simulink model "siWDqudong_FAN_MPC"  (R2024b)
settings: Solver=ode4  StartTime=0.0  StopTime=30  FixedStep=0.0005  RelTol=1e-3
undefined symbols (not defined in the file): MotorData, Q_beta_tune, Q_yaw_tune, R_alloc_tune, R_rate_tune, Road_Curvature_Map, Road_Mu_Map, Sim_Mu_Set, Sim_Vx_Set, Target_Speed_Map, W_util_tune
libraries: Solver_SF x1
(part 2 of 3)

== matlab function siWDqudong_FAN_MPC/Subsystem1/MATLAB Function2 ==
  settings: updateMethod=DISCRETE
  data: T_fl input; P_total_kW output; T_fr input; T_rl input; T_rr input; w_fl input; w_fr input; w_rl input; w_rr input; Map_Spd input; Map_Trq input; Map_Eff input; dt input; is_reset input; E_total_kWh output; P_avg_kW output
function [P_total_kW, E_total_kWh, P_avg_kW] = Calc_Energy_Internal_Map(...
    T_fl, T_fr, T_rl, T_rr, ...       
    w_fl, w_fr, w_rl, w_rr, ...       
    Map_Spd, Map_Trq, Map_Eff, ...    
    dt, is_reset)                     
%#codegen
% =========================================================================
% 全工况能耗计算器 v11.1 (最终版)
% [核心特性]
% 1. 完整覆盖驱动与制动回收双象限查表 (原样保留负转矩传入查表)。
% 2. 包含 35% 低扭效率兜底机制，避免除零或无穷大功率奇点，更贴合实际物理下限。
% 3. 包含车规级制动回收保护：低速 (<5 rad/s) 与低效 (<20%) 区间强制切断。
% =========================================================================
    persistent E_accumulated_J Total_Time_s
    if isempty(E_accumulated_J) || is_reset
        E_accumulated_J = 0;
        Total_Time_s = 0;
    end
    
    T_vec = [double(T_fl), double(T_fr), double(T_rl), double(T_rr)];
    w_vec = [double(w_fl), double(w_fr), double(w_rl), double(w_rr)];
    
    % --- ★ 轮毂电机物理与工程参数 ★ ---
    i_gear = 1.0; % 直驱轮毂电机减速比
    P_base_loss_W = 150.0; % 逆变器与控制器的基础待机损耗 (W)
    
    vec_x_rad = double(Map_Spd); 
    vec_y_nm  = double(Map_Trq); 
    mat_eff   = double(Map_Eff)';
    
    P_elec_W_vec = zeros(1, 4);
    
    for i = 1:4
        T_wheel = T_vec(i);     
        w_wheel_rads = w_vec(i);     
        
        % 1. 计算电机端工况
        % ★ 核心：速度取绝对值，扭矩保留正负号，以精确匹配四象限 Map 表！
        T_motor = T_wheel / i_gear; 
        w_motor_rads = abs(w_wheel_rads) * i_gear; 
        
        % 计算轮端机械功率 (驱动时为正，制动反拖时为负)
        P_mech_wheel = T_wheel * w_wheel_rads; 
        
        % 2. 极端静止/空转工况拦截
        if abs(w_wheel_rads) < 1.0
            % 车辆基本停稳，电机停止输出，彻底切断电能消耗
            P_elec = 0; 
        elseif abs(T_wheel) < 3.0 
            % 车辆滑行或该轮被上层分配 0 扭矩，仅消耗基础待机电量
            P_elec = P_base_loss_W; 
        else
            % 3. 正常工况：查表获取当前效率
            eff_raw = manual_interp2(vec_x_rad, vec_y_nm, mat_eff, w_motor_rads, T_motor);
            
            % 4. 驱动与制动能量流向计算
            if P_mech_wheel > 0
                % =========================================================
                % 【驱动耗电模式】
                % 引入 35% 的工程效率兜底，防止极低扭矩时的能耗被数学奇点无限放大
                % 消耗电功率 = (机械功率 / 效率) + 基础待机功耗
                % =========================================================
                eff_final = max(eff_raw, 0.35); 
                P_elec = (P_mech_wheel / eff_final) + P_base_loss_W;
                
            else
                % =========================================================
                % 【制动回收模式 (Regenerative Braking)】
                % P_mech_wheel 为负值
                % =========================================================
                if eff_raw < 0.20 || w_motor_rads < 5.0 
                    % 工程保护机制：低速域或极低效率域，强行切断激磁回收
                    % 避免开关损耗大于回收收益的现象
                    P_elec = P_base_loss_W; 
                else
                    % 物理能量守恒：
                    % 负的机械功率 * 效率 = 缩水的负电功率 (代表实际回充至母线的电量)
                    % 加上正的待机功耗，进一步减少了最终充入电池的能量
                    P_elec = (P_mech_wheel * eff_raw) + P_base_loss_W; 
                end
            end
        end
        % 记录单个车轮的总电功率
        P_elec_W_vec(i) = P_elec;
    end
    
    % --- 5. 整车能耗累加与统计 ---
    P_total_W = sum(P_elec_W_vec);       % 整车瞬时总功率 (W)
    P_total_kW = P_total_W / 1000;       % 整车瞬时总功率 (kW)
    
    % 焦耳积分 (J = W * s)
    E_accumulated_J = E_accumulated_J + P_total_W * double(dt);
    Total_Time_s = Total_Time_s + double(dt);
    
    % 转换为 kWh (1 kWh = 3.6e6 J)
    E_total_kWh = E_accumulated_J / 3.6e6;
    
    % 计算全历程平均功率
    if Total_Time_s > 1e-3
        P_avg_kW = (E_accumulated_J / Total_Time_s) / 1000;
    else
        P_avg_kW = 0;
    end
end

% ==== 手写双线性插值函数 (Bilinear Interpolation) ====
function val = manual_interp2(X, Y, Z, xq, yq)
    % 边界钳位保护
    xq_c = max(min(xq, X(end)), X(1));
    yq_c = max(min(yq, Y(end)), Y(1));
    
    % 寻找 X 轴索引
    idx_x = 1;
    for k = 1:length(X)-1
        if xq_c >= X(k) && xq_c <= X(k+1), idx_x = k; break; end
    end
    
    % 寻找 Y 轴索引
    idx_y = 1;
    for k = 1:length(Y)-1
        if yq_c >= Y(k) && yq_c <= Y(k+1), idx_y = k; break; end
    end
    
    x1 = X(idx_x); x2 = X(idx_x+1);
    y1 = Y(idx_y); y2 = Y(idx_y+1);
    
    % 归一化局部坐标
    if abs(x2-x1)<1e-9, u=0; else, u=(xq_c-x1)/(x2-x1); end
    if abs(y2-y1)<1e-9, v=0; else, v=(yq_c-y1)/(y2-y1); end
    
    % 四点提取
    f11 = Z(idx_y,   idx_x);
    f21 = Z(idx_y,   idx_x+1);
    f12 = Z(idx_y+1, idx_x);
    f22 = Z(idx_y+1, idx_x+1);
    
    % 双线性加权
    val = (1-v)*((1-u)*f11 + u*f21) + v*((1-u)*f12 + u*f22);
    
    if isnan(val), val = 0.01; end
end

== matlab function siWDqudong_FAN_MPC/Subsystem1/MATLAB Function17 ==
  data: Vx input; r_d output; delta_f input; mu input; m input; lf input; lr input; K_s output; r_ideal output; Kf0 input; Kr0 input; g input; r_limit output
function [r_d, K_s, r_ideal, r_limit] = ReferenceYawRate(Vx, delta_f, mu, m, lf, lr, Kf0, Kr0, g)
% =========================================================================
% 参考横摆角速度生成 (鲁棒增强版)
% 修复内容：低速奇点保护、物理极限柔性化、输出平滑
% =========================================================================

    % 1. 参数默认值与保护
    if nargin < 9, g = 9.81; end
    
    % 输入数据维度清洗 (强制转为标量 double)
    Vx_in = double(Vx(1));
    delta_in = double(delta_f(1));
    mu_in = double(mu(1));

    % 速度方向与绝对值处理
    Vx_sign = sign(Vx_in);
    if Vx_sign == 0, Vx_sign = 1; end
    Vx_abs = abs(Vx_in);
    
    % 基础防除零保护 (计算模型用)
    Vx_safe = max(Vx_abs, 0.5); 

    % =====================================================================
    % 2. 计算稳态增益 (Steady State Gain)
    % =====================================================================
    K_s = m / (2 * (lf + lr)^2) * (lr/Kf0 - lf/Kr0);

    % =====================================================================
    % 3. 计算理想横摆角速度 (Linear 2DOF Model)
    % =====================================================================
    % 分母：1 + K * V^2
    denom = (lf + lr) * (1 + K_s * Vx_safe^2);
    
    if abs(denom) < 0.1
        r_ideal = 0;
    else
        % r_ideal = (Vx / L(1+KV^2)) * delta
        r_ideal = (Vx_safe / denom) * delta_in * Vx_sign; 
    end

    % =====================================================================
    % 4. 计算物理极限 (【关键修复点】)
    % =====================================================================
    % 原公式：Limit = 0.85 * mu * g / Vx
    % 问题：当车辆甩尾速度掉到 1m/s 时，Limit 会变成 0.85*0.8*9.8/1 = 6.6 rad/s (380度/秒)
    % 修复：计算极限时，假设速度至少为 5m/s (虚拟速度钳位)
    % 逻辑：低速时侧向加速度其实达不到 mu*g，因为离心力不够，所以这样限制更符合物理
    
    Vx_for_limit = max(Vx_abs, 5.0); 
    
    % 计算理论上限
    r_limit_val = 0.85 * mu_in * g / Vx_for_limit;
    
    % 【双重保险】增加一个绝对硬限幅 (例如 1.5 rad/s ≈ 85 deg/s)
    % 防止任何情况下的数值爆炸
    r_limit_val = min(r_limit_val, 1.5);

    % =====================================================================
    % 5. 柔性限幅 (Saturation)
    % =====================================================================
    if r_ideal > r_limit_val
        r_d_raw = r_limit_val;
    elseif r_ideal < -r_limit_val
        r_d_raw = -r_limit_val;
    else
        r_d_raw = r_ideal;
    end

    % =====================================================================
    % 6. 强力滤波 (平滑输出)
    % =====================================================================
    persistent rd_prev
    if isempty(rd_prev), rd_prev = 0; end
    
    % 滤波系数：0.05 代表非常强的滤波 (响应慢，但稳)，如果觉得滞后太大可改为 0.1
    alpha_filter = 0.05; 
    
    r_d_smooth = (1 - alpha_filter) * rd_prev + alpha_filter * r_d_raw;
    
    % 更新记忆
    rd_prev = r_d_smooth;

    % =====================================================================
    % 7. 输出类型转换
    % =====================================================================
    r_d = double(r_d_smooth);
    r_ideal = double(r_ideal);
    r_limit = double(r_limit_val);
    
end

== matlab function siWDqudong_FAN_MPC/Subsystem1/MATLAB Function15 ==
  data: Vx_cmd input; Vx_act_raw input; T_total output; Ax_cmd input; m input; g input; r_e input; Kp input; Ki input; dt input; is_reset input; T_ff output; T_fb output; delta_steering input; Mu_in input; Curv_in input; Beta_in input; SI_in input
function [T_total, T_ff, T_fb] = Calc_Total_Demand_Torque( ...
    Vx_cmd, Vx_act_raw, Ax_cmd, ...
    m, g, r_e, ...
    Kp, Ki, dt, is_reset, delta_steering, Mu_in, ...
    Curv_in, Beta_in, SI_in)
%#codegen
% Fixed-speed longitudinal torque demand for closed-loop BO.
% Safety remains enforced by physical torque limits and downstream
% stability constraints; the controller does not silently lower Vx_cmd.

    persistent Vx_act_f Mu_f steer_f T_prev T_int Risk_f initialized

    if isempty(Vx_act_f) || is_reset
        Vx_act_f = double(Vx_act_raw);
        Mu_f = max(0.15,double(Mu_in(1)));
        steer_f = abs(double(delta_steering));
        T_prev = 0.0;
        T_int = 0.0;
        Risk_f = 0.0;
        initialized = false;
    end

    if dt <= 1e-5
        dt = 0.01;
    end

    Vx_cmd_use = max(0.0,double(Vx_cmd));
    Vx_act_raw_use = max(0.0,double(Vx_act_raw));
    Ax_cmd_use = double(Ax_cmd);

    alpha_v = 0.08;
    alpha_mu = 0.03;
    alpha_st = 0.10;
    Vx_act_f = (1.0-alpha_v)*Vx_act_f + alpha_v*Vx_act_raw_use;
    Mu_raw = max(0.15,double(Mu_in(1)));
    Mu_f = (1.0-alpha_mu)*Mu_f + alpha_mu*Mu_raw;
    steer_f = (1.0-alpha_st)*steer_f + alpha_st*abs(double(delta_steering));

    Vx_act = Vx_act_f;
    Mu_est = Mu_f;

    kappa_abs = abs(double(Curv_in(1)));
    beta_abs = abs(double(Beta_in(1)));
    SI_val = double(SI_in(1));
    ay_req = Vx_act*Vx_act*kappa_abs;
    ay_lim = max(Mu_est*g,0.10);
    ay_ratio = ay_req/ay_lim;

    R_ay = clamp((ay_ratio-0.78)/0.15,0.0,1.0);
    R_beta = clamp((beta_abs-0.045)/0.035,0.0,1.0);
    R_SI = clamp((SI_val-0.65)/0.35,0.0,1.0);
    R_st = clamp((steer_f-0.030)/0.040,0.0,1.0);
    Raw_Risk = max([R_ay,0.8*R_beta,0.6*R_SI,0.4*R_st]);

    if Raw_Risk >= Risk_f
        alpha_risk = 0.18;
    else
        alpha_risk = 0.06;
    end
    Risk_f = (1.0-alpha_risk)*Risk_f + alpha_risk*Raw_Risk;
    Risk_long = clamp(Risk_f,0.0,1.0);

    % Road-load feedforward is evaluated at the commanded speed.  Blending
    % it toward measured speed creates positive feedback for underspeed and
    % caused the old V5 controller to keep losing torque as Vx fell.
    Vx_ff = Vx_cmd_use;
    Cd = 0.30;
    Af = 2.8;
    rho = 1.206;
    f_roll = 0.015;
    if abs(Vx_ff) > 0.2
        sgn_v = sign(Vx_ff);
    else
        sgn_v = 0.0;
    end
    F_aero = 0.5*rho*Cd*Af*Vx_ff*Vx_ff*sgn_v;
    F_roll = m*g*f_roll*sgn_v;
    F_acc = m*Ax_cmd_use;
    T_ff = (F_aero+F_roll+F_acc)*r_e;

    % Symmetric PI speed hold.  Risk is not allowed to disable positive
    % feedback; an infeasible fixed-speed condition must fail explicitly.
    e = Vx_cmd_use-Vx_act;
    deadband = 0.02;
    if e > deadband
        e_ctrl = e-deadband;
    elseif e < -deadband
        e_ctrl = e+deadband;
    else
        e_ctrl = 0.0;
    end

    Kp_use = max(double(Kp),0.0);
    Ki_use = max(double(Ki),0.0);
    T_int_old = T_int;
    T_int = clamp(T_int+Ki_use*e_ctrl*dt,-80.0,160.0);
    T_fb = Kp_use*e_ctrl+T_int;

    T_max_limit = 1500.0*(Mu_est/0.85);
    T_min_limit = -800.0*(Mu_est/0.85);
    if Risk_long > 0.28
        T_max_limit = max(160.0,0.82*T_max_limit);
    end

    T_cmd = T_ff+T_fb;
    T_sat = clamp(T_cmd,T_min_limit,T_max_limit);

    % Conditional integration prevents windup at the physical limits.
    if (T_cmd > T_max_limit && e_ctrl > 0.0) || ...
       (T_cmd < T_min_limit && e_ctrl < 0.0)
        T_int = T_int_old;
        T_fb = Kp_use*e_ctrl+T_int;
        T_cmd = T_ff+T_fb;
        T_sat = clamp(T_cmd,T_min_limit,T_max_limit);
    end

    % Initialize at the physical feedforward demand instead of ramping from
    % zero torque while the vehicle already starts at the target speed.
    if ~initialized || is_reset
        T_prev = T_sat;
        initialized = true;
    end

    if Risk_long > 0.28
        dT_up_rate = 500.0;
        dT_dn_rate = 800.0;
    else
        dT_up_rate = 800.0;
        dT_dn_rate = 800.0;
    end
    dT_up = dT_up_rate*dt;
    dT_dn = dT_dn_rate*dt;
    dT = T_sat-T_prev;
    if dT > dT_up
        T_total = T_prev+dT_up;
    elseif dT < -dT_dn
        T_total = T_prev-dT_dn;
    else
        T_total = T_sat;
    end
    T_prev = T_total;
end

function y = clamp(x,lo,hi)
    y = max(min(x,hi),lo);
end

== matlab function siWDqudong_FAN_MPC/Subsystem1/MATLAB Function18 ==
  settings: updateMethod=DISCRETE  sampleTime=0.01
  data: Vx_target_input input; Vx_safe_cmd output; dt input; Ax_cmd_final output
function [Vx_safe_cmd, Ax_cmd_final] = Constant_Speed_Planner(Vx_target_input, dt)
    % Constant_Speed_Planner
    % 功能：生成恒定目标车速和加速度指令
    
    % ================= 1. 数据预处理 (维度安全锁) =================
    % 强制转换为 double
    temp_v = double(Vx_target_input);
    
    % 【关键修改】防止输入变成向量 [4x1]
    % 如果输入是向量，取第一个元素或取平均值，确保输出是标量 [1x1]
    if numel(temp_v) > 1
        target_v = mean(temp_v); % 或者 target_v = temp_v(1);
    else
        target_v = temp_v;
    end
    
    % 限幅保护
    if isnan(target_v)
        target_v = 0;
    end
    target_v = max(target_v, 0); 

    % ================= 2. 指令生成 =================
    Vx_safe_cmd = target_v;
    
    % 理论加速度设为0
    Ax_cmd_final = 0; 
    
    % (可选) 如果未来想用 dt 做平滑处理，可以在这里写逻辑
    % 目前 dt 虽然未被使用，但保留在输入端口没问题，不会报错
end

== matlab function siWDqudong_FAN_MPC/Subsystem1/MATLAB Function19 ==
  data: Beta input; Beta_dot input; Vx input; mu input; delta_f input; SI_Out output
function SI_Out = fcn_Calculate_SI(Beta, Beta_dot, Vx, mu, delta_f)
%#codegen
%
% ================================================================
% TVT Phase-Plane Stability Index
% 与原始 TVT_PhasePlane_Deliverable_2026-09-06 中
% TVT_StableBoundary.m 的联合拟合模型严格一致
%
% Inputs:
%   Beta      - 质心侧偏角 beta [rad]
%   Beta_dot  - 质心侧偏角速度 beta_dot [rad/s]
%   Vx        - 车辆纵向速度 [m/s]
%   mu        - 路面附着系数 [-]
%   delta_f   - 前轮转角 [rad]
%
% Output:
%   SI_Out    - 相平面稳定性指标
%
% 原始定义：
%
%   lower <= beta + A*beta_dot <= upper
%
%   center = k * delta_f
%   lower  = center - B
%   upper  = center + B
%
%   SI = abs(beta + A*beta_dot - center) / B
%
%   SI <= 1 : 位于拟合稳定区域内部
%   SI >  1 : 超出拟合稳定边界
%
% ================================================================


%% ================================================================
% 1. 原始联合拟合输入标准化参数
% ================================================================

MuCenter = 0.588775510204082;
MuScale  = 0.199025047136673;

VCenter  = 19.530612244898;
VScale   = 6.17488880067328;


%% ================================================================
% 2. 标准化输入
% ================================================================

mu_s = (mu - MuCenter) / MuScale;
v_s  = (Vx - VCenter) / VScale;


%% ================================================================
% 3. 原始联合拟合：A(V,mu)
%
% X6 =
% [1,
%  mu_s,
%  v_s,
%  mu_s^2,
%  mu_s*v_s,
%  v_s^2]
%
% 系数完全来自：
% phase_joint_fit_coefficients.csv
% ================================================================

a0 =  0.161558225154477;
a1 = -0.0467387963496101;
a2 =  0.0117445583275526;
a3 =  0.0102656813192654;
a4 =  0.000166133673754782;
a5 =  0.012427427190128;

A = ...
      a0 ...
    + a1 * mu_s ...
    + a2 * v_s ...
    + a3 * mu_s * mu_s ...
    + a4 * mu_s * v_s ...
    + a5 * v_s * v_s;


%% ================================================================
% 4. 原始联合拟合：半宽 B(V,mu)
%
% X9 =
% [1,
%  mu_s,
%  v_s,
%  mu_s^2,
%  mu_s*v_s,
%  v_s^2,
%  mu_s^2*v_s,
%  mu_s*v_s^2,
%  mu_s^2*v_s^2]
%
% 系数完全来自：
% phase_joint_fit_coefficients.csv
% ================================================================

b0 =  0.109427337783177;
b1 =  0.0142990282924419;
b2 = -0.0381098451846239;
b3 =  0.00694057641920019;
b4 = -0.00200034946269806;
b5 =  0.0266201953812123;
b6 =  0.0105740728277829;
b7 = -0.00475737528037003;
b8 = -0.00798511539344205;

mu_s2 = mu_s * mu_s;
v_s2  = v_s  * v_s;

B = ...
      b0 ...
    + b1 * mu_s ...
    + b2 * v_s ...
    + b3 * mu_s2 ...
    + b4 * mu_s * v_s ...
    + b5 * v_s2 ...
    + b6 * mu_s2 * v_s ...
    + b7 * mu_s * v_s2 ...
    + b8 * mu_s2 * v_s2;


%% ================================================================
% 5. 原始联合拟合：中心位置 C(delta_f)
%
% 原始模型：
% center = ShiftK * delta_rad
% ================================================================

ShiftK = 1.00429232124377;

center = ShiftK * delta_f;


%% ================================================================
% 6. 原始相平面稳定性指标
%
% 与 TVT_StableBoundary.m 完全相同：
%
% SI = abs(beta + A*beta_dot - center)/B
% ================================================================

SI_Out = abs(Beta + A * Beta_dot - center) / B;

end

== matlab function siWDqudong_FAN_MPC/Subsystem1/MATLAB Function23 ==
  data: Fy_fl input; Cf_eq output; Fy_fr input; Fy_rl input; Fy_rr input; Alpha_fl input; Alpha_fr input; Alpha_rl input; Alpha_rr input; Cf0 input; Cr0 input; Cr_eq output; Mu_Current input
function [Cf_eq, Cr_eq] = fcn_Calc_Equivalent_Stiffness_Filtered(...
    Fy_fl, Fy_fr, Fy_rl, Fy_rr, ...
    Alpha_fl, Alpha_fr, Alpha_rl, Alpha_rr, ...
    Cf0, Cr0, Mu_Current) % ★ 新增输入: 当前路面附着 Mu_Current
% =========================================================================
% 非线性侧偏刚度估算模块 (前馈预警 + 实时估算混合版)
% =========================================================================
    persistent Cf_prev Cr_prev
    if isempty(Cf_prev)
        Cf_prev = Cf0 * 2; 
        Cr_prev = Cr0 * 2;
    end
    
    % =====================================================================
    % ★ 核心新增：基于附着系数的前馈压制 (Feed-forward Penalty) ★
    % 当车进入冰雪路面时，不用等侧滑发生，直接从物理极限上压低标称刚度！
    % =====================================================================
    mu_nominal = 0.85;
    mu_real = max(min(double(Mu_Current(1)), 1.0), 0.1);
    % 计算附着衰减系数
    mu_ratio = mu_real / mu_nominal; 
    
    % 前馈修正后的基础刚度 (冰面上基础刚度会瞬间掉下来)
    Cf_base_dyn = (Cf0 * 2) * mu_ratio;
    Cr_base_dyn = (Cr0 * 2) * mu_ratio;

    Fy_front_sum = abs(Fy_fl + Fy_fr);
    Fy_rear_sum  = abs(Fy_rl + Fy_rr);
    Alpha_front_avg = abs(Alpha_fl + Alpha_fr) / 2.0;
    Alpha_rear_avg  = abs(Alpha_rl + Alpha_rr) / 2.0;
    
    alpha_deadzone = 0.0087; 
    
    if Alpha_front_avg > alpha_deadzone
        Cf_inst = Fy_front_sum / Alpha_front_avg;
    else
        Cf_inst = Cf_base_dyn; % 小角度时用前馈修正的刚度
    end
    
    if Alpha_rear_avg > alpha_deadzone
        Cr_inst = Fy_rear_sum / Alpha_rear_avg;
    else
        Cr_inst = Cr_base_dyn; % 小角度时用前馈修正的刚度
    end
    
    % ★ 限幅逻辑也要跟着附着系数前馈一起下降 ★
    Cf_min = Cf_base_dyn * 0.3;  Cf_max = Cf_base_dyn * 1.5;
    Cr_min = Cr_base_dyn * 0.3;  Cr_max = Cr_base_dyn * 1.5;
    
    Cf_target = max(min(Cf_inst, Cf_max), Cf_min);
    Cr_target = max(min(Cr_inst, Cr_max), Cr_min);
    
    % 为了应对附着突变，如果是从高附着到低附着（刚度需要暴降），加快滤波速度
    if Cf_target < Cf_prev
        lambda = 0.3; % 变滑了，降刚度要快！(0.05太慢了)
    else
        lambda = 0.05; % 恢复抓地力，慢慢升
    end
    
    Cf_filt = (1 - lambda) * Cf_prev + lambda * Cf_target;
    Cr_filt = (1 - lambda) * Cr_prev + lambda * Cr_target;
    
    Cf_prev = Cf_filt; Cr_prev = Cr_filt;
    Cf_eq = Cf_filt; Cr_eq = Cr_filt;
end

== matlab function siWDqudong_FAN_MPC/Subsystem1/MATLAB Function5 ==
  data: Vx input; Sx_fr output; Vy input; r input; omega_fr input; delta_f input; lf input; twf input; Re input; Sy_fr output; Vsx_fr output; Vsy_fr output
function [Sx_fr, Sy_fr, Vsx_fr, Vsy_fr] = Cal_UniTire_FullData_FR(Vx, Vy, r, omega_fr, delta_f, lf, twf, Re)
% Cal_UniTire_FullData_FR - 右前轮全参数计算

    % === 1. 运动学解算 ===
    % 右前轮：纵向 +lf, 横向 -twf/2 (右侧)
    % Vx修正: 右侧轮在左转(r>0)时线速度增加，所以是 + r*(twf/2)
    V_cx = Vx + r * (twf / 2);  
    V_cy = Vy + r * lf;         

    % === 2. 坐标旋转 (车轮坐标系) ===
    cos_d = cos(delta_f);
    sin_d = sin(delta_f);
    
    V_long = V_cx * cos_d + V_cy * sin_d;
    V_lat  = -V_cx * sin_d + V_cy * cos_d;

    % === 3. 计算滑移速度 (能耗用) ===
    V_wheel = omega_fr * Re;
    Vsx_fr = V_wheel - V_long; % 纵向滑移速度
    Vsy_fr = V_lat;            % 侧向滑移速度

    % === 4. 计算滑移率 (轮胎模型用) ===
    V_long_safe = max(abs(V_long), 1.0); 
    
    Sx_fr = Vsx_fr / V_long_safe;
    Sy_fr = -Vsy_fr / V_long_safe; % UniTire定义带负号

    % === 5. 限幅 ===
    Sx_fr = max(min(Sx_fr, 1.5), -1.5);
    Sy_fr = max(min(Sy_fr, 1.5), -1.5);
end

== matlab function siWDqudong_FAN_MPC/Subsystem1/MATLAB Function6 ==
  data: Vx input; Sx_rl output; Vy input; r input; omega_rl input; lr input; twr input; Re input; Sy_rl output; Vsx_rl output; Vsy_rl output
function [Sx_rl, Sy_rl, Vsx_rl, Vsy_rl] = Cal_UniTire_FullData_RL(Vx, Vy, r, omega_rl, lr, twr, Re)
% Cal_UniTire_FullData_RL - 左后轮全参数计算
% 注意：后轮默认无转向角 (delta = 0)

    % === 1. 运动学解算 ===
    % 左后轮：纵向 -lr, 横向 +twr/2 (左侧)
    % Vcx: 左侧减去横摆分量
    % Vcy: 后轴减去横摆分量 (Vy - r*lr)
    V_cx = Vx - r * (twr / 2);  
    V_cy = Vy - r * lr;         

    % === 2. 坐标旋转 (后轮 delta=0) ===
    % cos(0)=1, sin(0)=0，其实就是不用旋转
    V_long = V_cx;
    V_lat  = V_cy;

    % === 3. 计算滑移速度 (能耗用) ===
    V_wheel = omega_rl * Re;
    Vsx_rl = V_wheel - V_long; 
    Vsy_rl = V_lat;            

    % === 4. 计算滑移率 (轮胎模型用) ===
    V_long_safe = max(abs(V_long), 1.0); 
    
    Sx_rl = Vsx_rl / V_long_safe;
    Sy_rl = -Vsy_rl / V_long_safe;

    % === 5. 限幅 ===
    Sx_rl = max(min(Sx_rl, 1.5), -1.5);
    Sy_rl = max(min(Sy_rl, 1.5), -1.5);
end

== matlab function siWDqudong_FAN_MPC/Subsystem1/MATLAB Function7 ==
  data: Vx input; Sx_rr output; Vy input; r input; omega_rr input; lr input; twr input; Re input; Sy_rr output; Vsx_rr output; Vsy_rr output
function [Sx_rr, Sy_rr, Vsx_rr, Vsy_rr] = Cal_UniTire_FullData_RR(Vx, Vy, r, omega_rr, lr, twr, Re)
% Cal_UniTire_FullData_RR - 右后轮全参数计算
% 注意：后轮默认无转向角 (delta = 0)

    % === 1. 运动学解算 ===
    % 右后轮：纵向 -lr, 横向 -twr/2 (右侧)
    % Vcx: 右侧加上横摆分量
    % Vcy: 后轴减去横摆分量
    V_cx = Vx + r * (twr / 2);  
    V_cy = Vy - r * lr;         

    % === 2. 坐标旋转 (后轮 delta=0) ===
    V_long = V_cx;
    V_lat  = V_cy;

    % === 3. 计算滑移速度 (能耗用) ===
    V_wheel = omega_rr * Re;
    Vsx_rr = V_wheel - V_long; 
    Vsy_rr = V_lat;            

    % === 4. 计算滑移率 (轮胎模型用) ===
    V_long_safe = max(abs(V_long), 1.0); 
    
    Sx_rr = Vsx_rr / V_long_safe;
    Sy_rr = -Vsy_rr / V_long_safe;

    % === 5. 限幅 ===
    Sx_rr = max(min(Sx_rr, 1.5), -1.5);
    Sy_rr = max(min(Sy_rr, 1.5), -1.5);
end

== matlab function siWDqudong_FAN_MPC/Subsystem1/unitire轮胎力 ==
  data: Vx input; Vy input; r input; Sx_fl output; omega_fl input; delta_f input; lf input; twf input; Sy_fl output; Re input; Vsx_fl output; Vsy_fl output
function [Sx_fl, Sy_fl, Vsx_fl, Vsy_fl] = Cal_UniTire_FullData_FL(Vx, Vy, r, omega_fl, delta_f, lf, twf, Re)
% Cal_UniTire_FullData_FL - 左前轮全参数计算
% 输出: 
%   Sx, Sy: UniTire定义的滑移率 (无量纲) -> 用于查表或公式算力
%   Vsx, Vsy: 轮胎接地点滑移速度 (m/s) -> 用于 P = F * V 算能耗

    % === 1. 运动学解算：计算【轮心】在【车身坐标系】下的速度 ===
    % (左前轮：纵向 +lf, 横向 +twf/2)
    % 注意：横摆 r 对纵向速度的影响是 -r*y, 对横向速度的影响是 +r*x
    V_cx = Vx - r * (twf / 2);  
    V_cy = Vy + r * lf;         

    % === 2. 坐标旋转：转换到【车轮坐标系】 ===
    cos_d = cos(delta_f);
    sin_d = sin(delta_f);
    
    % V_long: 车轮滚动方向速度 (即纵向速度 Vx_wheel)
    % V_lat:  车轮侧向速度 (即侧向速度 Vy_wheel)
    V_long = V_cx * cos_d + V_cy * sin_d;
    V_lat  = -V_cx * sin_d + V_cy * cos_d;

    % === 3. 计算滑移速度 (能耗计算的核心) ===
    % 轮缘线速度
    V_wheel = omega_fl * Re;

    % 纵向滑移速度 (Vsx): 也就是大家常说的“滑移速度差”
    % 物理含义：轮胎接地点相对于地面的向后速度
    Vsx_fl = V_wheel - V_long; 

    % 侧向滑移速度 (Vsy): 
    % 物理含义：轮胎整体侧滑的速度
    Vsy_fl = V_lat; 

    % === 4. 计算滑移率 (UniTire 轮胎力模型的核心) ===
    % 分母保护：防止停车或低速时除零，导致仿真崩溃
    % 选取 max(abs(V_long), 1.0) 是为了在低速下保证数值稳定
    V_long_safe = max(abs(V_long), 1.0); 
    
    % --- 纵向滑移率 Sx ---
    % UniTire 定义: Sx = (V_wheel - V_long) / V_long
    % 等价于: Sx = Vsx / V_long
    Sx_fl = Vsx_fl / V_long_safe;

    % --- 侧向滑移率 Sy ---
    % UniTire 定义: Sy = - V_lat / V_long
    % 等价于: Sy = - Vsy / V_long
    % 注意：UniTire 的 Sy 定义通常带有负号 (对应 -tan(alpha))
    Sy_fl = -Vsy_fl / V_long_safe;

    % === 5. 物理限幅 (防止数值爆炸) ===
    % 仅对滑移率限幅，滑移速度(Vsx/Vsy)是物理真值，不要限幅！
    Sx_fl = max(min(Sx_fl, 1.5), -1.5);
    Sy_fl = max(min(Sy_fl, 1.5), -1.5);

end

== matlab function siWDqudong_FAN_MPC/Subsystem1/侧偏角计算 ==
  data: Vx input; alpha_fl output; Vy input; r input; delta_f_rad input; lf input; lr input; twf input; twr input; alpha_fr output; alpha_rl output; alpha_rr output
function [alpha_fl, alpha_fr, alpha_rl, alpha_rr] = Block2_SlipAngle(...
    Vx, Vy, r, delta_f_rad, lf, lr, twf, twr)
% =========================================================================
% BLOCK2_SLIPANGLE - 四轮侧偏角计算 (纯弧度版)
% 
% [关键设置]
% 1. 输入 delta_f_rad 必须是【弧度】(您已在外部转换好)。
% 2. 输出 alpha 均为【弧度】。
% 3. 符号修正：采用 (转向角 - 速度角) 逻辑，确保左转产生正滑移角。
% =========================================================================

    % 1. 速度方向保护 (防止分母为0)
    Vx_safe = max(abs(Vx), 0.1) * sign(Vx); 
    if Vx_safe == 0, Vx_safe = 0.1; end
    
    % 2. 轮心速度解算 (运动学公式)
    % -----------------------------------------------------------
    % 左前轮 (Left-Front)
    Vx_fl = Vx_safe - (r * twf) / 2;
    Vy_fl = Vy + (r * lf);
    
    % 右前轮 (Right-Front)
    Vx_fr = Vx_safe + (r * twf) / 2;
    Vy_fr = Vy + (r * lf);
    
    % 左后轮 (Left-Rear)
    Vx_rl = Vx_safe - (r * twr) / 2;
    Vy_rl = Vy - (r * lr);
    
    % 右后轮 (Right-Rear)
    Vx_rr = Vx_safe + (r * twr) / 2;
    Vy_rr = Vy - (r * lr);
    
    % 3. 侧偏角计算 (核心修正)
    % -----------------------------------------------------------
    % 公式：Alpha = 转向角 - 速度矢量角
    % atan2 计算结果天然是弧度，与您的输入 delta_f_rad (弧度) 直接相减
    
    % 左前
    theta_fl = atan2(Vy_fl, Vx_fl);
    alpha_fl = delta_f_rad - theta_fl; 
    
    % 右前
    theta_fr = atan2(Vy_fr, Vx_fr);
    alpha_fr = delta_f_rad - theta_fr;
    
    % 左后 (后轮转向角 delta = 0)
    theta_rl = atan2(Vy_rl, Vx_rl);
    alpha_rl = 0 - theta_rl; 
    
    % 右后
    theta_rr = atan2(Vy_rr, Vx_rr);
    alpha_rr = 0 - theta_rr; 

    % 4. 输出清理
    % -----------------------------------------------------------
    % 确保输出为实数
    alpha_fl = real(alpha_fl);
    alpha_fr = real(alpha_fr);
    alpha_rl = real(alpha_rl);
    alpha_rr = real(alpha_rr);
    
    % [注意] 输出的是弧度！
    % 如果接下来的刚度模块或轮胎模块需要弧度，直接连线即可。
    % 后面【千万不要】再接那个 pi/180 的 Gain 模块了！
end

== matlab function siWDqudong_FAN_MPC/Subsystem1/横纵向附着系数 ==
  data: road_condition input; mu_x output; slip_ratio input; mu_y output
function [mu_x, mu_y] = FrictionCoefficientLookup(road_condition, slip_ratio)
% 基于路面条件和滑移率的摩擦系数查表
% 输入: road_condition - 路面类型 (1=冰面, 2=雪面, 3=湿沥青, 4=干沥青)
%       slip_ratio - 当前滑移率（可选，用于动态调整）

    switch road_condition
        case 1 % 冰面（论文实验条件）
            mu_x = 0.2;
            mu_y = 0.18;  % 横向摩擦系数通常略低
            
        case 2 % 雪面
            mu_x = 0.3;
            mu_y = 0.25;
            
        case 3 % 湿沥青
            mu_x = 0.5;
            mu_y = 0.45;
            
        case 4 % 干沥青
            mu_x = 0.85;
            mu_y = 0.80;
            
        otherwise
            mu_x = 0.8;
            mu_y = 0.75;
    end
    
    % 可选：基于滑移率的动态调整（Burckhardt模型简化版）
    if nargin > 1
        % 典型摩擦系数-滑移率曲线（冰面）
        if road_condition == 1
            optimal_slip = 0.08;  % 冰面最佳滑移率
            if slip_ratio > optimal_slip
                % 超过最佳滑移率后摩擦系数下降
                mu_x = mu_x * (1 - 0.5 * (slip_ratio - optimal_slip));
                mu_y = mu_y * (1 - 0.6 * (slip_ratio - optimal_slip));
            end
        end
    end
end

== matlab function siWDqudong_FAN_MPC/Subsystem1/MATLAB Function1 ==
  data: Sx_fl input; Sy_fl input; Fx_fl output; Fz_fl input; mu_x input; mu_y input; Kx input; Ky input; Fy_fl output; Fbar_x_fl output; Fbar_y_fl output; E input
function [Fx_fl, Fy_fl, Fbar_x_fl, Fbar_y_fl] = Cal_Force_FL(Sx_fl, Sy_fl, Fz_fl, mu_x, mu_y, Kx, Ky, E)
% Cal_Force_FL - 左前轮 UniTire (完整版)
% 输入:
% Sx_fl, Sy_fl: 纵横向滑移率
% Fz_fl: 垂向载荷 (N)
% mu_x, mu_y: 纵向/横向 峰值附着系数 (例如 1.0, 0.9)
% Kx, Ky: 轮胎纵向/横向刚度 (N/1)
% E: UniTire 曲率因子 (通常 0.5~1.0，决定峰值后的形状)

% 0. 数据保护
Fz_safe = max(Fz_fl, 100); % 防止 Fz=0 报错
% 1. 计算相对滑移率 (Relative Slip, phi)
% 分别针对纵向和横向极限进行归一化
% phi_x = (Kx * Sx) / (mu_x * Fz)
phi_x = (Kx * abs(Sx_fl)) / (mu_x * Fz_safe);
phi_y = (Ky * abs(Sy_fl)) / (mu_y * Fz_safe);
% 合成相对滑移率 (摩擦椭圆耦合核心)
phi = sqrt(phi_x^2 + phi_y^2);

% 2. 计算总归一化力 (F_bar)
% UniTire 经验公式: F_bar = 1 - exp(-phi - E * phi^2)
% 这里的 E 就是您要找回的曲率因子
if phi < 1e-6
F_bar = 0;
else
F_bar = 1 - exp(-phi - E * phi^2);
end

% 3. 分解回横纵向 (分配方向)
% Fbar_x 是归一化分量 (0~1)
if phi < 1e-6
Fbar_x_fl = 0;
Fbar_y_fl = 0;
else
Fbar_x_fl = F_bar * (phi_x / phi);
Fbar_y_fl = F_bar * (phi_y / phi);
end

% 4. 计算真实物理力 (Physical Force, N)
% 必须乘回各自方向的极限力 (mu * Fz)
Max_Force_X = mu_x * Fz_safe;
Max_Force_Y = mu_y * Fz_safe;
Fx_abs = Fbar_x_fl * Max_Force_X;
Fy_abs = Fbar_y_fl * Max_Force_Y;

% 5. 恢复符号
Fx_fl = sign(Sx_fl) * Fx_abs;
Fy_fl = sign(Sy_fl) * Fy_abs;
end

== matlab function siWDqudong_FAN_MPC/Subsystem1/MATLAB Function8 ==
  data: Sx_rl input; Sy_rl input; Fx_rl output; Fz_rl input; mu_x input; mu_y input; Kx input; Ky input; Fy_rl output; Fbar_x_rl output; Fbar_y_rl output; E input

function [Fx_rl, Fy_rl, Fbar_x_rl, Fbar_y_rl] = Cal_Force_RL(Sx_rl, Sy_rl, Fz_rl, mu_x, mu_y, Kx, Ky, E)
% Cal_Force_RL - 左后轮 UniTire (完整版)

Fz_safe = max(Fz_rl, 100);

% 1. 相对滑移率
phi_x = (Kx * abs(Sx_rl)) / (mu_x * Fz_safe);
phi_y = (Ky * abs(Sy_rl)) / (mu_y * Fz_safe);
phi = sqrt(phi_x^2 + phi_y^2);

% 2. 总归一化力
if phi < 1e-6
F_bar = 0;
else
F_bar = 1 - exp(-phi - E * phi^2);
end

% 3. 分量分配
if phi < 1e-6
Fbar_x_rl = 0;
Fbar_y_rl = 0;
else
Fbar_x_rl = F_bar * (phi_x / phi);
Fbar_y_rl = F_bar * (phi_y / phi);
end

% 4. 真实力
Fx_rl = sign(Sx_rl) * (Fbar_x_rl * (mu_x * Fz_safe));
Fy_rl = sign(Sy_rl) * (Fbar_y_rl * (mu_y * Fz_safe));
end

== matlab function siWDqudong_FAN_MPC/Subsystem1/MATLAB Function9 ==
  data: Sx_fr input; Sy_fr input; Fx_fr output; Fz_fr input; mu_x input; mu_y input; Kx input; Ky input; Fy_fr output; Fbar_x_fr output; Fbar_y_fr output; E input
function [Fx_fr, Fy_fr, Fbar_x_fr, Fbar_y_fr] = Cal_Force_FR(Sx_fr, Sy_fr, Fz_fr, mu_x, mu_y, Kx, Ky, E)
% Cal_Force_FR - 右前轮 UniTire (完整版)

Fz_safe = max(Fz_fr, 100);

% 1. 相对滑移率
phi_x = (Kx * abs(Sx_fr)) / (mu_x * Fz_safe);
phi_y = (Ky * abs(Sy_fr)) / (mu_y * Fz_safe);
phi = sqrt(phi_x^2 + phi_y^2);

% 2. 总归一化力 (带 E)
if phi < 1e-6
F_bar = 0;
else
F_bar = 1 - exp(-phi - E * phi^2);
end

% 3. 分量分配
if phi < 1e-6
Fbar_x_fr = 0;
Fbar_y_fr = 0;
else
Fbar_x_fr = F_bar * (phi_x / phi);
Fbar_y_fr = F_bar * (phi_y / phi);
end

% 4. 真实力 (乘回 mu*Fz)
Fx_fr = sign(Sx_fr) * (Fbar_x_fr * (mu_x * Fz_safe));
Fy_fr = sign(Sy_fr) * (Fbar_y_fr * (mu_y * Fz_safe));
end

== matlab function siWDqudong_FAN_MPC/Subsystem1/MATLAB Function10 ==
  data: Sx_rr input; Sy_rr input; Fx_rr output; Fz_rr input; mu_x input; mu_y input; Kx input; Ky input; E input; Fy_rr output; Fbar_x_rr output; Fbar_y_rr output
function [Fx_rr, Fy_rr, Fbar_x_rr, Fbar_y_rr] = Cal_Force_RR(Sx_rr, Sy_rr, Fz_rr, mu_x, mu_y, Kx, Ky, E)
% Cal_Force_RR - 右后轮 UniTire (完整版)

Fz_safe = max(Fz_rr, 100);

% 1. 相对滑移率
phi_x = (Kx * abs(Sx_rr)) / (mu_x * Fz_safe);
phi_y = (Ky * abs(Sy_rr)) / (mu_y * Fz_safe);
phi = sqrt(phi_x^2 + phi_y^2);

% 2. 总归一化力
if phi < 1e-6
F_bar = 0;
else
F_bar = 1 - exp(-phi - E * phi^2);
end

% 3. 分量分配
if phi < 1e-6
Fbar_x_rr = 0;
Fbar_y_rr = 0;
else
Fbar_x_rr = F_bar * (phi_x / phi);
Fbar_y_rr = F_bar * (phi_y / phi);
end

% 4. 真实力
Fx_rr = sign(Sx_rr) * (Fbar_x_rr * (mu_x * Fz_safe));
Fy_rr = sign(Sy_rr) * (Fbar_y_rr * (mu_y * Fz_safe));
end

== matlab function siWDqudong_FAN_MPC/Subsystem1/MATLAB Function14 ==
  data: NN_Weights output; Vx_kmh input; Vref_kmh input; Mu_current input; Kappa_current input; Mu_preview input; Kappa_preview input
function NN_Weights = Call_NN_Mapper(Vx_kmh, Vref_kmh, Mu_current, Kappa_current, Mu_preview, Kappa_preview)
%#codegen
% =========================================================================
% Reference-speed-aware risk-preserving 4D BO-BPNN weight mapper
%
% BPNN input:
%   X_NN = [V_NN, mu_risk, kappa_risk, D_safe]^T
%
% Key idea:
%   1) The BPNN still uses a 4D input.
%   2) The first input is not the raw measured speed, but a risk-preserving
%      speed feature V_NN.
%   3) In low-risk conditions, V_NN follows the measured speed Vx.
%   4) In high-risk conditions, V_NN approaches the reference-speed-aware
%      risk speed, but is capped to avoid excessive conservativeness.
% =========================================================================

    NN_Weights = zeros(5, 1, 'double');

    %% ============================================================
    % 0. Tunable parameters
    % ============================================================
    Ts_ctrl = 0.01;          % Control sampling time, s

    D_low  = 0.50;           % Risk-gate lower threshold
    D_high = 0.70;           % Risk-gate upper threshold

    DeltaV_cap = 10.0;        % km/h, max allowed gap between V_NN and Vx
                             % If SI is still high, try 10~12.
                             % If speed drops too much, try 5~6.

    lambda_D = 0.10;         % 1/s, linear decay rate of D_safe

    %% ============================================================
    % 1. Signal reading and protection
    % ============================================================
    Vx = double(Vx_kmh(1));
    if ~isfinite(Vx)
        Vx = 60.0;
    end
    Vx = min(max(Vx, 0.0), 120.0);

    Vref = double(Vref_kmh(1));
    if ~isfinite(Vref) || Vref <= 1.0
        Vref = Vx;
    end
    Vref = min(max(Vref, 0.0), 120.0);

    Mu_c = double(Mu_current(1));
    Mu_p = double(Mu_preview(1));

    if ~isfinite(Mu_c) || Mu_c <= 0
        Mu_c = 0.85;
    end

    if ~isfinite(Mu_p) || Mu_p <= 0
        Mu_p = Mu_c;
    end

    mu_risk = min(Mu_c, Mu_p);
    mu_risk = max(mu_risk, 0.10);

    Kappa_c = abs(double(Kappa_current(1)));
    Kappa_p = abs(double(Kappa_preview(1)));

    if ~isfinite(Kappa_c)
        Kappa_c = 0.0;
    end

    if ~isfinite(Kappa_p)
        Kappa_p = 0.0;
    end

    kappa_risk = max(Kappa_c, Kappa_p);

    %% ============================================================
    % 2. Reference-speed-aware risk gate
    % ============================================================
    D_ref = ((Vref / 3.6)^2 * kappa_risk) / max(mu_risk * 9.81, 1e-6);
    D_ref = min(max(D_ref, 0.0), 1.0);

    gamma = (D_ref - D_low) / max(D_high - D_low, 1e-6);
    gamma = min(max(gamma, 0.0), 1.0);

    %% ============================================================
    % 3. Risk-preserving speed feature
    % ============================================================
    V_risk = min(Vref, Vx + DeltaV_cap);
    V_risk = max(V_risk, Vx);

    V_NN = (1.0 - gamma) * Vx + gamma * V_risk;
    V_NN = min(max(V_NN, 0.0), 120.0);

    %% ============================================================
    % 4. Risk calculation with linear peak-hold decay
    % ============================================================
    D_raw = ((V_NN / 3.6)^2 * kappa_risk) / max(mu_risk * 9.81, 1e-6);
    D_raw = min(max(D_raw, 0.0), 1.0);

    persistent D_safe_prev;
    if isempty(D_safe_prev)
        D_safe_prev = 0.0;
    end

    D_safe = max(D_raw, D_safe_prev - lambda_D * Ts_ctrl);
    D_safe = min(max(D_safe, 0.0), 1.0);
    D_safe_prev = D_safe;

    %% ============================================================
    % 5. BPNN forward inference
    % ============================================================
    X_in = [V_NN; mu_risk; kappa_risk; D_safe];

    NN_out = BPNN_Core_Ultimate_Res(X_in);

    %% ============================================================
    % 6. Physical baseline and NN residual reconstruction
    % ============================================================
    base_R = 4.5 - 3.5 * D_safe;
    base_W = 1.0 + 3.5 * D_safe;

    res_R_alloc = max(-2.0, min(2.0, NN_out(3)));
    res_W_slip  = max(-2.0, min(3.0, NN_out(5)));

    log_R_alloc_nn = base_R + res_R_alloc;
    log_W_slip_nn  = base_W + res_W_slip;

    log_Q_beta_nn = NN_out(1);
    log_Q_yaw_nn  = NN_out(2);
    log_R_rate_nn = NN_out(4) - 0.5 * (D_safe^2);

    %% ============================================================
    % 7. Risk-dependent safety envelope for W_slip
    % ============================================================
    envelope_W = -16.2 * (D_safe^2) + 32.8 * D_safe - 11.6;
    envelope_W = max(0.0, envelope_W);

    log_W_slip_final = max(log_W_slip_nn, envelope_W);

    %% ============================================================
    % 8. High-risk priority shift
    % ============================================================
    risk_barrier = max(0.0, D_safe - 0.7) / 0.3;
    risk_barrier = min(max(risk_barrier, 0.0), 1.0);

    penalty_others = 1.0 * risk_barrier;

    log_R_alloc_final = log_R_alloc_nn - penalty_others;
    log_R_rate_final  = log_R_rate_nn  - penalty_others;
    log_Q_beta_final  = log_Q_beta_nn  - penalty_others;
    log_Q_yaw_final   = log_Q_yaw_nn   - penalty_others;

    %% ============================================================
    % 9. Log-domain bounds
    % ============================================================
    log_W_slip_final  = max(-1.0, min(6.0, log_W_slip_final));
    log_R_alloc_final = max(-1.0, min(6.0, log_R_alloc_final));
    log_R_rate_final  = max(-1.0, min(6.0, log_R_rate_final));
    log_Q_beta_final  = max(-1.0, min(6.0, log_Q_beta_final));
    log_Q_yaw_final   = max(-1.0, min(6.0, log_Q_yaw_final));

    %% ============================================================
    % 10. Log-domain filtering
    % ============================================================
    logW_raw = [
        log_Q_beta_final;
        log_Q_yaw_final;
        log_R_alloc_final;
        log_R_rate_final;
        log_W_slip_final
    ];

    persistent logW_prev;
    if isempty(logW_prev)
        logW_prev = logW_raw;
    end

    alpha = 0.1 + 0.3 * D_safe;
    alpha = min(max(alpha, 0.05), 0.45);

    logW_filt = (1.0 - alpha) * logW_prev + alpha * logW_raw;
    logW_prev = logW_filt;

    %% ============================================================
    % 11. Exponential reconstruction
    % ============================================================
    NN_Weights(1) = 10^logW_filt(1);   % Q_beta
    NN_Weights(2) = 10^logW_filt(2);   % Q_r
    NN_Weights(3) = 10^logW_filt(3);   % R_alloc
    NN_Weights(4) = 10^logW_filt(4);   % R_rate
    NN_Weights(5) = 10^logW_filt(5);   % W_slip
end

== matlab function siWDqudong_FAN_MPC/Subsystem1/MATLAB Function16 ==
  data: Fx_fl input; Px_fl output; Fy_fl input; Sx_fl input; Sy_fl input; Vx input; Vy input; r input; delta_f input; lf input; twf input; Py_fl output
function [Px_fl, Py_fl] = Cal_Power_FL(Fx_fl, Fy_fl, Sx_fl, Sy_fl, Vx, Vy, r, delta_f, lf, twf)
% Cal_Power_FL - 左前轮横纵向滑移功耗计算
% 基于 UniTire 模型定义的滑移率和力进行能量损耗计算
%
% 输入:
%   Fx_fl, Fy_fl: 轮胎纵向/横向力 (N) [来自力计算模块]
%   Sx_fl, Sy_fl: 轮胎纵向/横向滑移率 [来自滑移率模块]
%   Vx, Vy: 质心速度 (m/s)
%   r: 横摆角速度 (rad/s)
%   delta_f: 前轮转角 (rad)
%   lf: 质心到前轴距离 (m)
%   twf: 前轮距 (m)
%
% 输出:
%   Px_fl: 纵向滑移功耗 (W)
%   Py_fl: 横向滑移功耗 (W)

    % 1. 重新计算轮心纵向速度 V_long (用于将滑移率还原为滑移速度)
    % 运动学：左前轮位置 (+lf, +twf/2)
    V_cx = Vx - r * (twf / 2); % 减去横摆线速度
    V_cy = Vy + r * lf;        % 加上横摆线速度

    % 坐标旋转到车轮坐标系
    cos_d = cos(delta_f);
    sin_d = sin(delta_f);
    
    % V_long 是车轮滚动方向的速度
    V_long = V_cx * cos_d + V_cy * sin_d;
    
    % 保护：防止低速除零或噪声，与滑移率模块保持一致的基准
    V_long_abs = max(abs(V_long), 1.0);

    % 2. 计算纵向滑移功耗 (Longitudinal Slip Power)
    % 公式: Power = Force * Sliding_Velocity
    % Sliding_Velocity_X = Sx * V_long
    % 取绝对值因为功耗总是正值 (能量耗散)
    Px_fl = abs(Fx_fl * (Sx_fl * V_long_abs));

    % 3. 计算横向滑移功耗 (Lateral Slip Power)
    % 公式: Power = Force * Lateral_Sliding_Velocity
    % 根据 UniTire 定义: Sy = -V_lat / V_long  => V_lat = -Sy * V_long
    % 同样取绝对值
    Py_fl = abs(Fy_fl * (Sy_fl * V_long_abs));

end

== matlab function siWDqudong_FAN_MPC/Subsystem1/MATLAB Function21 ==
  data: Fx input; E_long_total output; E_lat_total output; Fy input; Vsx input; Vsy input; dt input
function [E_long_total, E_lat_total] = Cal_Slip_Energy_Internal(Fx, Fy, Vsx, Vsy, dt)
    % Cal_Slip_Energy_Internal - 计算并内部积分横纵向滑移总能耗
    % 输出: 
    %   E_long_total: 四个车轮累计消耗的纵向摩擦能量 (Joules)
    %   E_lat_total:  四个车轮累计消耗的侧向摩擦能量 (Joules)

    % === 1. 定义持久变量 (用于在函数内部存储“上一时刻”的能量) ===
    persistent E_long_acc E_lat_acc

    % === 2. 初始化 (仅在仿真第一步执行) ===
    if isempty(E_long_acc)
        E_long_acc = 0;
        E_lat_acc = 0;
    end

    % === 3. 计算瞬时总功率 (Watts) ===
    % 绝对值 abs() 确保无论是驱动/制动还是左转/右转，都在耗能
    % .* 是对应元素相乘，sum 是把四个车轮的功率加在一起
    
    P_long_inst = sum(abs(Fx .* Vsx)); % 四轮纵向总瞬时功率
    P_lat_inst  = sum(abs(Fy .* Vsy)); % 四轮侧向总瞬时功率

    % === 4. 内部积分 (欧拉积分法) ===
    % 能量(J) = 旧能量 + 功率(W) * 时间步长(s)
    
    E_long_acc = E_long_acc + P_long_inst * dt;
    E_lat_acc  = E_lat_acc  + P_lat_inst  * dt;

    % === 5. 输出当前累计能耗 ===
    E_long_total = E_long_acc;
    E_lat_total  = E_lat_acc;

end

== matlab function siWDqudong_FAN_MPC/Subsystem1/MATLAB Function22 ==
  data: Fx_fr input; Px_fr output; Fy_fr input; Sx_fr input; Sy_fr input; Vx input; Vy input; r input; delta_f input; lf input; twf input; Py_fr output
function [Px_fr, Py_fr] = Cal_Power_FR(Fx_fr, Fy_fr, Sx_fr, Sy_fr, Vx, Vy, r, delta_f, lf, twf)
% Cal_Power_FR - 右前轮横纵向滑移功耗计算
% 注意：运动学计算中的符号与左轮不同

    % 1. 重新计算轮心纵向速度 V_long
    % 运动学：右前轮位置 (+lf, -twf/2 => 右侧通常定义为y轴负方向或正方向，此处依据您之前的代码逻辑)
    % 依据之前的逻辑：右轮横摆分量是 Vx + r*(twf/2)
    V_cx = Vx + r * (twf / 2); 
    V_cy = Vy + r * lf;

    % 坐标旋转
    cos_d = cos(delta_f);
    sin_d = sin(delta_f);
    
    V_long = V_cx * cos_d + V_cy * sin_d;
    V_long_abs = max(abs(V_long), 1.0);

    % 2. 纵向滑移功耗
    Px_fr = abs(Fx_fr * (Sx_fr * V_long_abs));

    % 3. 横向滑移功耗
    Py_fr = abs(Fy_fr * (Sy_fr * V_long_abs));

end

== matlab function siWDqudong_FAN_MPC/Subsystem1/MATLAB Function24 ==
  data: Fx_rl input; Px_rl output; Fy_rl input; Sx_rl input; Sy_rl input; Vx input; Vy input; r input; lr input; twr input; Py_rl output
function [Px_rl, Py_rl] = Cal_Power_RL(Fx_rl, Fy_rl, Sx_rl, Sy_rl, Vx, Vy, r, lr, twr)
% Cal_Power_RL - 左后轮横纵向滑移功耗计算
% 后轮无转向角 delta，故 V_long 直接等于 V_cx

    % 1. 重新计算轮心纵向速度 V_long
    % 运动学：左后轮位置 (-lr, +twr/2)
    % 左轮：Vx - r * (twr/2)
    V_long = Vx - r * (twr / 2);
    
    % 后轮无转向，无需坐标旋转，V_long 即为轮心纵向速度
    V_long_abs = max(abs(V_long), 1.0);

    % 2. 纵向滑移功耗
    Px_rl = abs(Fx_rl * (Sx_rl * V_long_abs));

    % 3. 横向滑移功耗
    Py_rl = abs(Fy_rl * (Sy_rl * V_long_abs));

end

== matlab function siWDqudong_FAN_MPC/Subsystem1/MATLAB Function25 ==
  data: Fx_rr input; Px_rr output; Fy_rr input; Sx_rr input; Sy_rr input; Vx input; Vy input; r input; lr input; twr input; Py_rr output
function [Px_rr, Py_rr] = Cal_Power_RR(Fx_rr, Fy_rr, Sx_rr, Sy_rr, Vx, Vy, r, lr, twr)
% Cal_Power_RR - 右后轮横纵向滑移功耗计算

    % 1. 重新计算轮心纵向速度 V_long
    % 运动学：右后轮位置 (-lr, -twr/2)
    % 右轮：Vx + r * (twr/2)
    V_long = Vx + r * (twr / 2);
    
    V_long_abs = max(abs(V_long), 1.0);

    % 2. 纵向滑移功耗
    Px_rr = abs(Fx_rr * (Sx_rr * V_long_abs));

    % 3. 横向滑移功耗
    Py_rr = abs(Fy_rr * (Sy_rr * V_long_abs));

end

== matlab function siWDqudong_FAN_MPC/Subsystem1/MATLAB Function20 ==
  data: Fx_fl input; Td output; Fx_fr input; Fx_rl input; Fx_rr input; r_e input; T_fl output; T_fr output; T_rl output; T_rr output
function[Td,T_fl,T_fr,T_rl,T_rr]  = calc_total_demand_torque(Fx_fl, Fx_fr, Fx_rl, Fx_rr, r_e)
% 计算总需求转矩Td
% 输入参数：
%   Fx_fl, Fx_fr, Fx_rl, Fx_rr: 四个车轮的纵向力 (N)，驱动为正，制动为负
%   r_e: 轮胎有效半径 (m)
% 输出参数：
%   Td: 总需求转矩 (Nm)

% 计算总纵向力
F_x_total = Fx_fl + Fx_fr + Fx_rl + Fx_rr;

% 总需求转矩 = 总纵向力 × 轮胎有效半径
T_fl = Fx_fl* r_e;
T_fr = Fx_fr* r_e;
T_rl = Fx_rl* r_e;
T_rr = Fx_rr* r_e;
Td = F_x_total * r_e;

% 数值稳定性处理（可选，若需避免极端值）
Td = real(Td);
end
